simulink model "Simulador_PID"  (R2024b)
settings: Solver=VariableStepAuto  StartTime=0.0  StopTime=2  RelTol=1e-3
values from neighbouring files (symbols this model uses):
  Kd = [Kd1;Kd1;Kd1]    [PROYECTO_D.m]
  Ki = [Ki1;Ki2;Ki3]    [PROYECTO_D.m]
  Kp = [Kp1;Kp1;Kp1]    [PROYECTO_D.m]
undefined symbols (not defined in the file or in its folder): CinematicaInversa
settings Model: Creator=aleja  LastModifiedBy=aleja
settings DataIOCC: ReturnWorkspaceOutputs=off

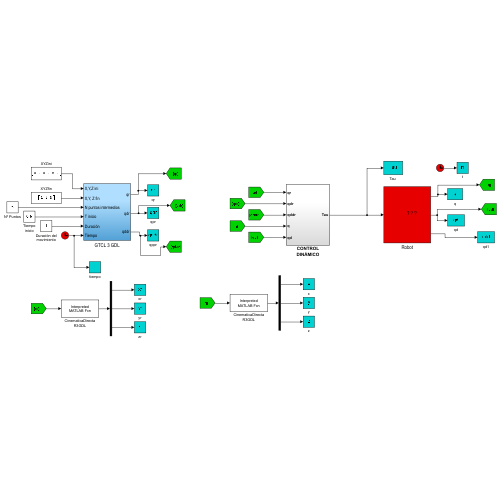
[thumbnail: Simulink's stored preview of the top-level diagram]
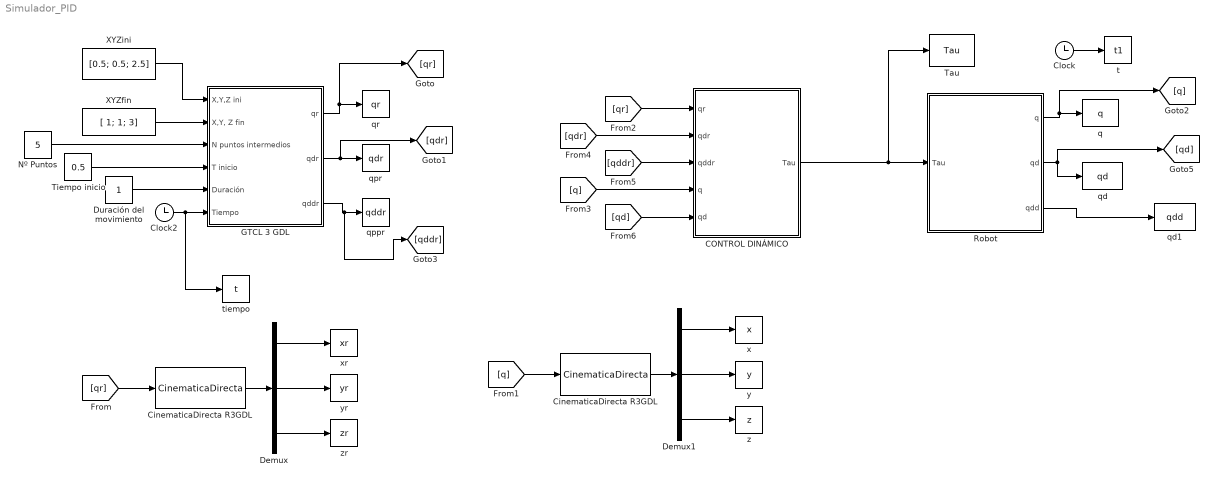
== system Simulador_PID ==
  CONTROL DINÁMICO : Subsystem
  CinematicaDirecta R3GDL : MATLABFcn  MATLABFcn=CinematicaDirecta  OutputDimensions=3
  "CinematicaDirecta R3GDL " : MATLABFcn  MATLABFcn=CinematicaDirecta  OutputDimensions=3
  Clock : Clock
  Clock2 : Clock
  Demux : Demux  Outputs=3
  Demux1 : Demux  Outputs=3
  Duración del movimiento : Constant
  GTCL 3 GDL : Subsystem
  Nº Puntos : Constant  Value=5
  Robot : Subsystem
      mask Display: image('R3GDL.jpg')
  "Tau " : ToWorkspace  VariableName=Tau  SampleTime=-1
  Tiempo inicio : Constant  Value=0.5
  XYZfin : Constant  Value=[ 1; 1; 3]
  XYZini : Constant  Value=[0.5; 0.5; 2.5]
  q : ToWorkspace  VariableName=q  SampleTime=-1
  qd : ToWorkspace  VariableName=qd  SampleTime=-1
  qd1 : ToWorkspace  VariableName=qdd  SampleTime=-1
  qppr : ToWorkspace  VariableName=qddr  SampleTime=-1
  qpr : ToWorkspace  VariableName=qdr  SampleTime=-1
  qr : ToWorkspace  VariableName=qr  SampleTime=-1
  t : ToWorkspace  VariableName=t1  SampleTime=-1
  tiempo : ToWorkspace  VariableName=t  SampleTime=-1
  x : ToWorkspace  VariableName=x  SampleTime=-1
  xr : ToWorkspace  VariableName=xr  SampleTime=-1
  y : ToWorkspace  VariableName=y  SampleTime=-1
  yr : ToWorkspace  VariableName=yr  SampleTime=-1
  z : ToWorkspace  VariableName=z  SampleTime=-1
  zr : ToWorkspace  VariableName=zr  SampleTime=-1
  wires:
  Demux/2 -> yr/1
  GTCL 3 GDL/3(qddr) -> [qddr], qppr/1
  GTCL 3 GDL/2(qdr) -> [qdr], qpr/1
  "CinematicaDirecta R3GDL "/1 -> Demux1/1
  Demux1/2 -> y/1
  Duración del movimiento/1 -> GTCL 3 GDL/5(Duración)
  [q] -> "CinematicaDirecta R3GDL "/1
  [qddr] -> CONTROL DINÁMICO/3(qddr)
  [q] -> CONTROL DINÁMICO/4(q)
  Demux/3 -> zr/1
  [qr] -> CONTROL DINÁMICO/1(qr)
  Nº Puntos/1 -> GTCL 3 GDL/3(N puntos intermedios)
  [qdr] -> CONTROL DINÁMICO/2(qdr)
  Demux/1 -> xr/1
  XYZfin/1 -> GTCL 3 GDL/2("X,Y, Z fin")
  GTCL 3 GDL/1(qr) -> qr/1, [qr]
  Demux1/3 -> z/1
  XYZini/1 -> GTCL 3 GDL/1(X,Y,Z ini)
  Clock2/1 -> tiempo/1, GTCL 3 GDL/6(Tiempo)
  [qd] -> CONTROL DINÁMICO/5(qd)
  CinematicaDirecta R3GDL/1 -> Demux/1
  [qr] -> CinematicaDirecta R3GDL/1
  Demux1/1 -> x/1
  Tiempo inicio/1 -> GTCL 3 GDL/4(T inicio)
  Robot/1(q) -> [q], q/1
  Robot/2(qd) -> qd/1, [qd]
  Clock/1 -> t/1
  Robot/3(qdd) -> qd1/1
  CONTROL DINÁMICO/1(Tau) -> "Tau "/1, Robot/1(Tau)

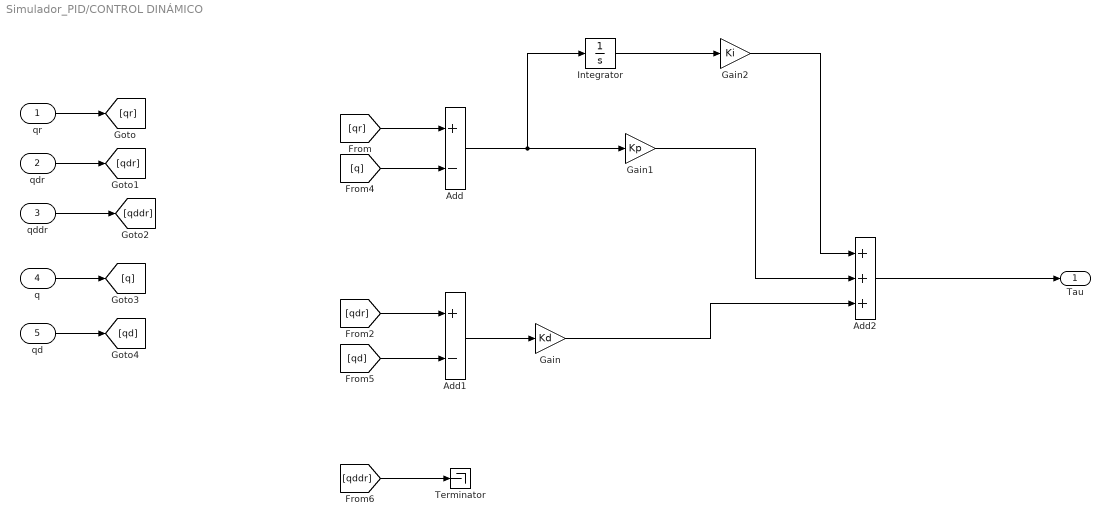
== system Simulador_PID/CONTROL DINÁMICO ==
  qr : Inport
  qdr : Inport  Port=2
  qddr : Inport  Port=3
  q : Inport  Port=4
  qd : Inport  Port=5
  Add : Sum  Inputs=+-
  Add1 : Sum  Inputs=+-
  Add2 : Sum  Inputs=+++
  Gain : Gain  Gain=Kd
  Gain1 : Gain  Gain=Kp
  Gain2 : Gain  Gain=Ki
  Integrator : Integrator
  Terminator : Terminator
  Tau : Outport
  wires:
  qr/1 -> [qr]
  qdr/1 -> [qdr]
  qddr/1 -> [qddr]
  q/1 -> [q]
  qd/1 -> [qd]
  [qr] -> Add/1
  [q] -> Add/2
  [qddr] -> Terminator/1
  [qd] -> Add1/2
  [qdr] -> Add1/1
  Add/1 -> Integrator/1, Gain1/1
  Add1/1 -> Gain/1
  Gain/1 -> Add2/3
  Gain1/1 -> Add2/2
  Add2/1 -> Tau/1
  Integrator/1 -> Gain2/1
  Gain2/1 -> Add2/1

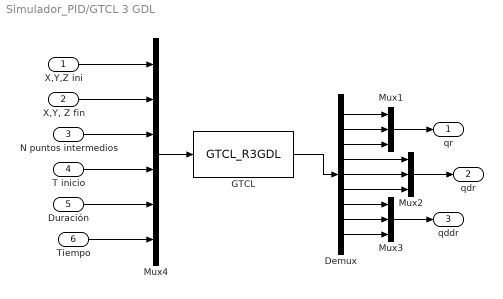
== system Simulador_PID/GTCL 3 GDL ==
  X,Y,Z ini : Inport
  "X,Y, Z fin" : Inport  Port=2
  N puntos intermedios : Inport  Port=3
  T inicio : Inport  Port=4
  Duración : Inport  Port=5
  Tiempo : Inport  Port=6
  Demux : Demux  Outputs=9
  GTCL : MATLABFcn  MATLABFcn=GTCL_R3GDL  OutputDimensions=9
  Mux1 : Mux  Inputs=3
  Mux2 : Mux  Inputs=3
  Mux3 : Mux  Inputs=3
  Mux4 : Mux  Inputs=6
  qr : Outport
  qdr : Outport  Port=2
  qddr : Outport  Port=3
  wires:
  Mux1/1 -> qr/1
  Mux4/1 -> GTCL/1
  X,Y,Z ini/1 -> Mux4/1
  "X,Y, Z fin"/1 -> Mux4/2
  N puntos intermedios/1 -> Mux4/3
  T inicio/1 -> Mux4/4
  Duración/1 -> Mux4/5
  Tiempo/1 -> Mux4/6
  GTCL/1 -> Demux/1
  Demux/1 -> Mux1/1
  Demux/2 -> Mux1/2
  Demux/3 -> Mux1/3
  Mux2/1 -> qdr/1
  Demux/4 -> Mux2/1
  Demux/5 -> Mux2/2
  Demux/6 -> Mux2/3
  Mux3/1 -> qddr/1
  Demux/7 -> Mux3/1
  Demux/8 -> Mux3/2
  Demux/9 -> Mux3/3

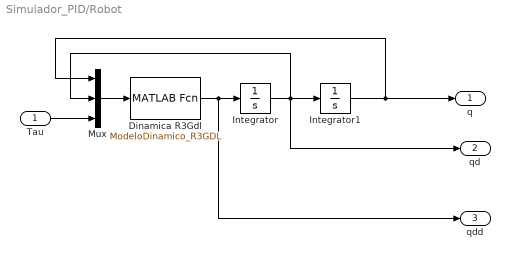
== system Simulador_PID/Robot ==
  Tau : Inport
  Dinamica R3Gdl : MATLABFcn  MATLABFcn=ModeloDinamico_R3GDL  OutputDimensions=3
  Integrator : Integrator  InitialCondition=[0;0;0];
  Integrator1 : Integrator  InitialCondition=CinematicaInversa([0.5; 0; 0.5])
  Mux : Mux  Inputs=3
  q : Outport
  qd : Outport  Port=2
  qdd : Outport  Port=3
  wires:
  Mux/1 -> Dinamica R3Gdl/1
  Dinamica R3Gdl/1 -> qdd/1, Integrator/1
  Integrator/1 -> Integrator1/1, qd/1, Mux/2
  Integrator1/1 -> q/1, Mux/1
  Tau/1 -> Mux/3
